simulink model "M9_NonLinearModel"  (Simulink 9.3)
settings: Solver=VariableStepAuto  StartTime=0.0  StopTime=10.0  RelTol=1e-3
undefined symbols (not defined in the file): Cg, Cs, k, kc, kg, kr, SelectIn, Ta, u0
settings Model: Creator=liguang  LastModifiedBy=炸酱面
settings DataIOCC: SaveFormat=Dataset  SignalLoggingSaveFormat=Dataset  ReturnWorkspaceOutputs=on
settings OptimizationCC: LifeSpan=auto
settings DebuggingCC: UnderspecifiedInitializationDetection=Simplified  MergeDetectMultiDrivingBlocksExec=error  FcnCallInpInsideContextMsg=error  SFUnexpectedBacktrackingDiag=error  SFNoUnconditionalDefaultTransitionDiag=error  SFExecutionAtInitializationDiag=warning  ArithmeticOperatorsInVariantConditions=error
settings HardwareCC: ProdBitPerPointer=64  ProdBitPerSizeT=64  ProdBitPerPtrDiffT=64  ProdLargestAtomicFloat=Float  ProdIntDivRoundTo=Zero  ProdEndianess=LittleEndian  ProdWordSize=64  ProdHWDeviceType=Intel->x86-64 (Windows64)
settings ModelReferenceCC: PropagateSignalLabelsOutOfModel=on
settings SFSimCC: SimUseLocalCustomCode=on
settings RTWCC: RTWUseLocalCustomCode=on
settings CodeAppCC: StateflowObjectComments=off
settings GRTTargetCC: TargetLangStandard=C99 (ISO)  CombineOutputUpdateFcns=on  GRTInterface=off
settings ConfigComp: CovMetricSettings=dwe  CovHtmlReporting=off  CovSaveCumulativeToWorkspaceVar=off  CovSaveSingleToWorkspaceVar=off  CovExternalEMLEnable=on

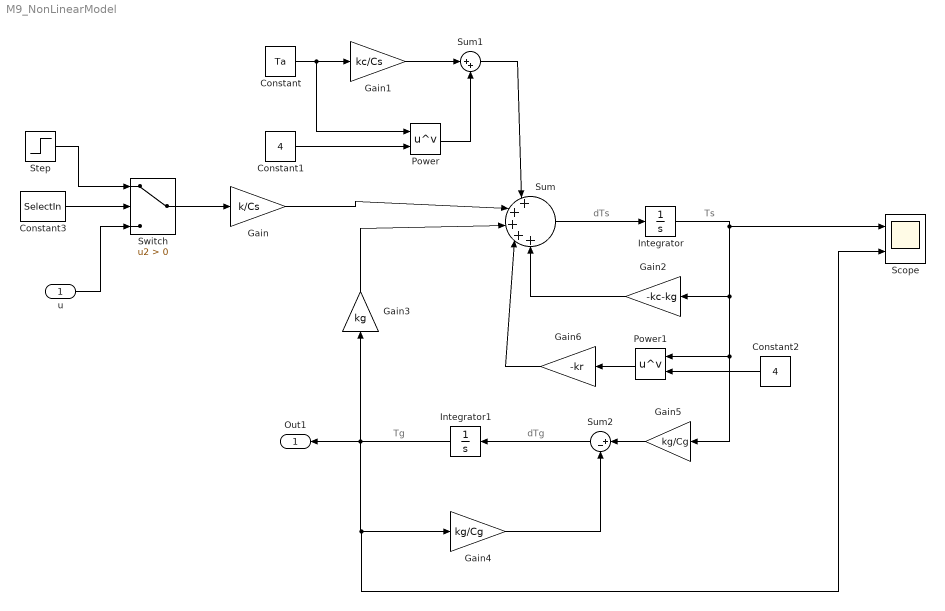
== system M9_NonLinearModel ==
  note: dTg
  note: Tg
  note: Ts
  note: dTs
  "u " : Inport
  Constant : Constant  Value=Ta
  Constant1 : Constant  Value=4
  Constant2 : Constant  Value=4
  Constant3 : Constant  Value=SelectIn
  Gain : Gain  Gain=k/Cs
  Gain1 : Gain  Gain=kc/Cs
  Gain2 : Gain  Gain=-kc-kg
  Gain3 : Gain  Gain=kg
  Gain4 : Gain  Gain=kg/Cg
  Gain5 : Gain  Gain=kg/Cg
  Gain6 : Gain  Gain=-kr
  Integrator : Integrator
  Integrator1 : Integrator
  Power : Math  Operator=pow  SaturateOnIntegerOverflow=on
  Power1 : Math  Operator=pow  SaturateOnIntegerOverflow=on
  Scope : Scope  NumInputPorts=2
  Step : Step  After=u0  SampleTime=0
  Sum : Sum  Inputs=|+|+|+|+|+
  Sum1 : Sum  Inputs=|++
  Sum2 : Sum  Inputs=|+-
  Switch : Switch  Criteria=u2 > Threshold
  Out1 : Outport
  wires:
  Gain/1 -> Sum/2
  Constant/1 -> Power/1, Gain1/1
  Gain1/1 -> Sum1/1
  Power/1 -> Sum1/2
  Sum1/1 -> Sum/1
  Sum/1 -> Integrator/1
  Integrator/1 -> Scope/1, Gain5/1, Power1/1, Gain2/1
  Gain2/1 -> Sum/5
  Constant1/1 -> Power/2
  Constant2/1 -> Power1/2
  Gain3/1 -> Sum/3
  Sum2/1 -> Integrator1/1
  Gain4/1 -> Sum2/2
  Gain5/1 -> Sum2/1
  Power1/1 -> Gain6/1
  Gain6/1 -> Sum/4
  "u "/1 -> Switch/3
  Switch/1 -> Gain/1
  Step/1 -> Switch/1
  Constant3/1 -> Switch/2
  Integrator1/1 -> Out1/1, Gain3/1, Scope/2, Gain4/1
